simulink model "dyn_pid_control_sim"  (R2019b)
settings: Solver=FixedStepAuto  StartTime=0.0  StopTime=63.05  FixedStep=h  RelTol=1e-3
values from neighbouring files (symbols this model uses):
  h = 0.1    [Example_9_Tracking_Delta_Input_Formulation.m]    (also in dyn_dist_mpc_control.m = 0.01; dyn_mpc_control.m = 0.01; dyn_pid_control.m = 0.01; init.m = 0.05)
  Kd = 5.6913    [dyn_pid_control.m]    (also in pid_control.m = 40.883)
  Ki = 1.9187    [dyn_pid_control.m]    (also in pid_control.m = 1.644)
  Kp = 23.086    [dyn_pid_control.m]    (also in pid_control.m = 34.562)
  N = 13.595    [pid_control.m]
libraries: simulink x1
settings Model: Creator=faaizz  LastModifiedBy=faaizz
settings SFSimCC: CustomCodeUndefinedFunction=UseInterfaceOnly

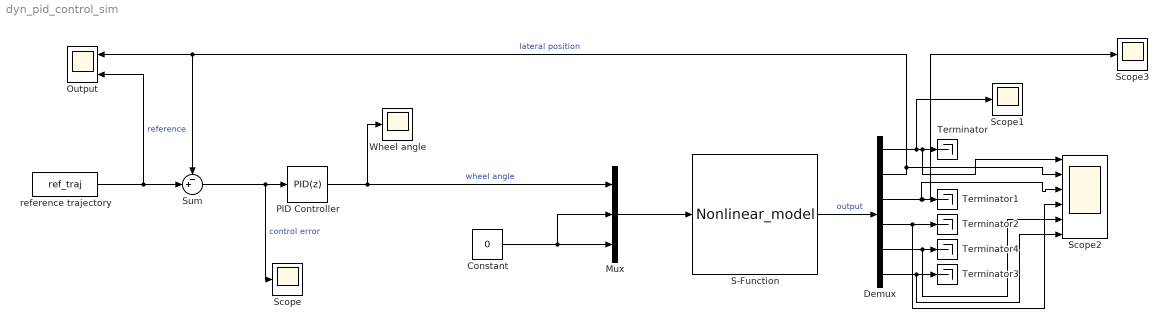
== system dyn_pid_control_sim ==
  Constant : Constant  Value=0
  Demux : Demux  Outputs=6
  Mux : Mux  Inputs=3
  Output : Scope  NumInputPorts=2
  PID Controller : simulink/Continuous/PID Controller  Controller=PID  Form=Parallel  TimeDomain=Discrete-time  SampleTime=h  IntegratorMethod=Forward Euler  FilterMethod=Forward Euler  ControllerParametersSource=internal  P=Kp*2  I=Kd*2  D=Ki  UseFilter=on  N=N  TunerSelectOption=Transfer Function Based (PID Tuner App)  InitialConditionSource=internal  InitialConditionForIntegrator=0  InitialConditionForFilter=0  DifferentiatorICPrevScaledInput=0  ExternalReset=none  TrackingMode=off  Kt=1  LimitOutput=off  UpperSaturationLimit=inf  LowerSaturationLimit=-inf  LinearizeAsGain=on  AntiWindupMode=none  Kb=1  POutMin=[]  POutMax=[]  IOutMin=[]  IOutMax=[]  DOutMin=[]  DOutMax=[]  NOutMin=[]  NOutMax=[]  SumOutMin=[]  SumOutMax=[]  SaturationOutMin=[]  SaturationOutMax=[]  PParamMin=[]  PParamMax=[]  IParamMin=[]  IParamMax=[]  DParamMin=[]  DParamMax=[]  NParamMin=[]  NParamMax=[]  KbParamMin=[]  KbParamMax=[]  KtParamMin=[]  KtParamMax=[]  KbOutMin=[]  KbOutMax=[]  KtOutMin=[]  KtOutMax=[]  IntegratorOutMin=[]  IntegratorOutMax=[]  FilterOutMin=[]  FilterOutMax=[]  SumI1OutMin=[]  SumI1OutMax=[]  SumI2OutMin=[]  SumI2OutMax=[]  SumI3OutMin=[]  SumI3OutMax=[]  SumI4OutMin=[]  SumI4OutMax=[]  SumDOutMin=[]  SumDOutMax=[]  DifferentiatorOutMin=[]  DifferentiatorOutMax=[]  FilterDiffOutCoefMin=[]  FilterDiffOutCoefMax=[]  ReciprocalOutMin=[]  ReciprocalOutMax=[]  SumDenOutMin=[]  SumDenOutMax=[]  SumNumOutMin=[]  SumNumOutMax=[]  DivideOutMin=[]  DivideOutMax=[]  IntegratorContinuousStateAttributes=''  IntegratorStateMustResolveToSignalObject=off  IntegratorRTWStateStorageClass=Auto  FilterContinuousStateAttributes=''  FilterStateMustResolveToSignalObject=off  FilterRTWStateStorageClass=Auto  ParallelPVariant=InternalParameters  IdealPVariant=Disabled  IVariant=InternalParameters  DVariant=InternalParameters  IntegratorVariant=Discrete  SatVariant=Disabled  AWVariant=Passthrough  PCopyVariant=Disabled  TRVariant=Disabled  FdbkBlocksVariant=Forward  IdealPFdbkVariant=Disabled  SatFdbkVariant=Disabled  DerivativeFilterVariant=ForwardEulerFilter  NVariant=InternalParameters  NCopyVariant=Disabled  FilterICVariant=InternalICsFilter  IntegratorICVariant=InternalICs  ExternalResetVariant=Disabled  TRSumVariant=Passthrough  SumFdbkVariant=Disabled  SumVariant=Sum_PID
  S-Function : S-Function  FunctionName=Nonlinear_model  SFunctionDeploymentMode=off  EnableBusSupport=off
  Scope : Scope
  Scope1 : Scope
  Scope2 : Scope  NumInputPorts=6
  Scope3 : Scope
  Sum : Sum  Inputs=-+|
  Terminator{,1..4} (5 alike) : Terminator
  Wheel angle : Scope
  reference trajectory : FromWorkspace  VariableName=ref_traj  SampleTime=0  OutputAfterFinalValue=Setting to zero
  wires:
  reference trajectory/1 -> Sum/2, Output/2  "reference"
  Sum/1 -> Scope/1, PID Controller/1  "control error"
  Constant/1 -> Mux/3, Mux/2
  Demux/2 -> Scope2/2, Sum/1, Output/1  "lateral position"
  S-Function/1 -> Demux/1  "output"
  Demux/3 -> Scope3/1, Terminator1/1, Scope2/3
  Demux/1 -> Scope1/1, Scope2/1, Terminator/1
  PID Controller/1 -> Mux/1, Wheel angle/1  "wheel angle"
  Demux/6 -> Scope2/6, Terminator3/1
  Mux/1 -> S-Function/1
  Demux/4 -> Scope2/4, Terminator2/1
  Demux/5 -> Scope2/5, Terminator4/1
